simulink library "ADRC_Toolbox"  (R2024a)
settings: Solver=VariableStepAuto  StartTime=0.0  StopTime=10.0  RelTol=1e-3
undefined symbols (not defined in the file or in its folder): build_robot_screw, ToolGroup, ToolSet, Ts, x0
libraries: $bdroot x14, simulink x7
(part 1 of 2)
settings Model: Creator=91015  LastModifiedBy=Chenfei Wang
settings SolverCC: AlgebraicLoopSolver=TrustRegion
settings DebuggingCC: UnconnectedInputMsg=warning  UnconnectedOutputMsg=warning  UnconnectedLineMsg=warning
settings ModelReferenceCC: EnableRefExpFcnMdlSchedulingChecks=on
settings SFSimCC: CustomCodeUndefinedFunction=UseInterfaceOnly
settings RTWCC: GPUComputeCapability=3.5  DLArmComputeVersion=19.05

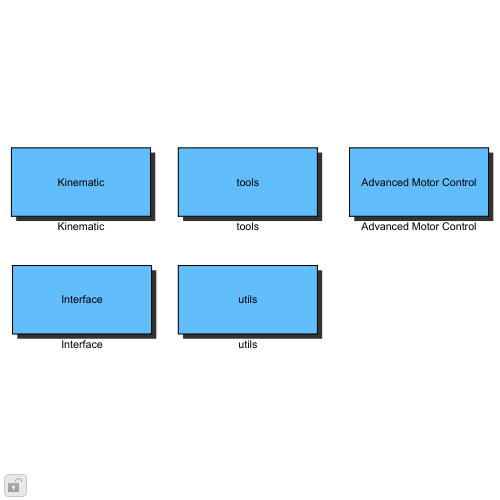
[thumbnail: Simulink's stored preview of the top-level diagram]
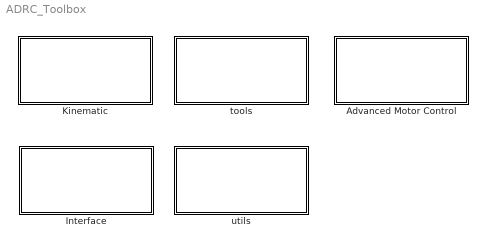
== system ADRC_Toolbox ==
  Advanced Motor Control : Subsystem  mask(tools){}
      mask Display: disp(get_param(gcb,'name'))
  Interface : Subsystem
      mask Display: disp(get_param(gcb,'name'))
  Kinematic : Subsystem
      mask Display: disp(get_param(gcb,'name'))
  tools : Subsystem  mask(tools){}
      mask Display: disp(get_param(gcb,'name'))
  utils : Subsystem  mask(tools){}
      mask Display: disp(get_param(gcb,'name'))

== system ADRC_Toolbox/Advanced Motor Control ==
  Basic : Subsystem
      mask Display: disp(get_param(gcb,'name'))
  Controller : Subsystem
      mask Display: disp(get_param(gcb,'name'))
  TD : Subsystem
      mask Display: disp(get_param(gcb,'name'))

== system ADRC_Toolbox/Interface ==
  note: encoder与 physical接口
  SC PC concat : Subsystem
  Tool Select : Subsystem
  allocateAllHands : MATLAB Function  TreatAsAtomicUnit=on
  checkToolTypeMatched : MATLAB Function  TreatAsAtomicUnit=on
  encoder2physical_PC : MATLAB Function  TreatAsAtomicUnit=on
  encoder2physical_SC : MATLAB Function  TreatAsAtomicUnit=on
  physical2encoder_PC : MATLAB Function  TreatAsAtomicUnit=on
  physical2encoder_SC : MATLAB Function  TreatAsAtomicUnit=on

== system ADRC_Toolbox/Kinematic ==
  Forward Kinematic : Subsystem  mask{ScrewObj=build_robot_screw, source_idx=0, target_idx=5}
      mask init:
      | ScrewObjName = get_param(gcb, 'ScrewObj');
      mask DialogControl DescGroupVar Prompt: Forward Kinematic
      mask DialogControl DescTextVar Prompt: 正向运动学,根据ScrewObj对象计算变换矩阵
      mask Display:
      | color('blue')
      | text(0.99, 0.99, ScrewObjName, 'horizontalAlignment', 'right', 'verticalAlignment','top');
      | 
      | color('black')
      | SourceText = ['Source: ' get_param(gcb,'source_idx')];
      | TargetText = ['Target: ' get_param(gcb,'target_idx')];
      | DescText = [SourceText newline TargetText];
      | text(0.5, 0.05, DescText, 'Interpreter', 'tex',  'horizontalAlignment', 'center','verticalAlignment','bottom');
      | 
      | color('black')
      | DescText = ['T' get_param(gcb,'source_idx') get_param(gcb,'target_idx')];
      | text(0.5, 0.8, DescText, 'Interpreter', 'tex',  'horizontalAlignment', 'center','verticalAlignment','bottom');
      | 
      | 
      | color('black')
      | port_label('input', 1, 'Config')
      | port_label('output', 1, 'Transform')
  Inverse Kinematic : Subsystem  mask{ScrewObj=build_robot_screw, Eomg=1e-5, Ev=1e-5, Lambda=0.2}
      mask init:
      | ScrewObjName = get_param(gcb, 'ScrewObj');
      mask DialogControl DescGroupVar Prompt: Inverse Kinematic
      mask DialogControl DescTextVar Prompt: 逆向运动学,给定T(相对base),使用LM算法求解
      mask Display:
      | color('blue')
      | text(0.99, 0.99, ScrewObjName, 'horizontalAlignment', 'right', 'verticalAlignment','top');
      | 
      | 
      | 
      | color('black')
      | port_label('input', 1, 'T')
      | port_label('input', 2, 'InitialGuass')
      | port_label('output', 1, 'theta')
      | port_label('output', 2, 'success')

== system ADRC_Toolbox/tools ==
  Clamp Tmatrix : MATLAB Function  TreatAsAtomicUnit=on
  Knife Tmatrix : MATLAB Function  TreatAsAtomicUnit=on
  Normal Tool Tmatrix : MATLAB Function  TreatAsAtomicUnit=on
  NormalTool_T2 : MATLAB Function  TreatAsAtomicUnit=on
  Scope Tmatrix : MATLAB Function  TreatAsAtomicUnit=on
  Screenangle2T : MATLAB Function  TreatAsAtomicUnit=on
  Stapler Tmatrix : MATLAB Function  TreatAsAtomicUnit=on
  ToolSet Select : Subsystem

== system ADRC_Toolbox/utils ==
  note: 错误代码
  Error Merge : Subsystem
  Error Store Memery : DataStoreMemory  DataStoreName=ErrorMemery  ReadBeforeWriteMsg=warning  WriteAfterWriteMsg=warning  WriteAfterReadMsg=warning  ShowAdditionalParam=off  OutDataTypeStr=uint16  Dimensions=1
  Tform2Vec : Subsystem
      mask Display:
      | color('black')
      | port_label('input', 1, 'T')
      | port_label('output', 1, 'Eul_ZYX')
      | port_label('output', 2, 'p')
  Tform2p : MATLAB Function  TreatAsAtomicUnit=on

== system ADRC_Toolbox/Advanced Motor Control/Basic ==
  Discrete State space with reset : Subsystem
      mask Display:
      | % port_label('input', 1, 'u')
      | % port_label('input', 2, 'A')
      | % port_label('input', 3, 'B')
      | % port_label('input', 4, 'C')
      | % port_label('input', 5, 'D')
      | % port_label('input', 6, 'x0')
      | % port_label('output', 1, 'y')
      | % port_label('output', 2, 'x')
      | % port_label('output', 3, 'dx')
      | 
      | text(0.5,0.65,'x_{k+1} = A x_k + B u_k',...
      |    'horizontalAlignment', 'center','texmode','on')
      | text(0.5,0.45,'y_k = C x_k + D u_k',...
      |    'horizontalAlignment', 'center','texmode','on')
      | text(0.5,0.25,'x0 with reset',...
      |    'horizontalAlignment', 'center','texmode','on')
  ODE4 Continue State space : Subsystem  mask{Ts=Ts}
      mask Display:
      | % port_label('input', 1, 'u')
      | % port_label('input', 2, 'A')
      | % port_label('input', 3, 'B')
      | % port_label('input', 4, 'C')
      | % port_label('input', 5, 'D')
      | % port_label('input', 6, 'x0')
      | % port_label('output', 1, 'y')
      | % port_label('output', 2, 'x')
      | % port_label('output', 3, 'dx')
      | 
      | text(0.5,0.65,'dx = A x + B u',...
      |    'horizontalAlignment', 'center','texmode','on')
      | text(0.5,0.45,'y = C x + D u',...
      |    'horizontalAlignment', 'center','texmode','on')
      | text(0.5,0.25,'x0 with reset',...
      |    'horizontalAlignment', 'center','texmode','on')
  State space with reset : Subsystem
      mask Display:
      | % port_label('input', 1, 'u')
      | % port_label('input', 2, 'A')
      | % port_label('input', 3, 'B')
      | % port_label('input', 4, 'C')
      | % port_label('input', 5, 'D')
      | % port_label('input', 6, 'x0')
      | % port_label('output', 1, 'y')
      | % port_label('output', 2, 'x')
      | % port_label('output', 3, 'dx')
      | 
      | text(0.5,0.65,'dx = A x + B u',...
      |    'horizontalAlignment', 'center','texmode','on')
      | text(0.5,0.45,'y = C x + D u',...
      |    'horizontalAlignment', 'center','texmode','on')
      | text(0.5,0.25,'x0 with reset',...
      |    'horizontalAlignment', 'center','texmode','on')

== system ADRC_Toolbox/Advanced Motor Control/Controller ==
  note: support code generation
  2nd order Discrete LADRC : Subsystem  mask{Ts=1e-3}
      mask prompts: Ts "Sampling Time"
  2nd order LADRC : Subsystem
  2nd order MC-ADRC : Subsystem  mask{a1=0}
      mask Display:
      | text(0.5,0.5,'ddx+a_1dx=b(u-f_{ext})',...
      |    'horizontalAlignment', 'center','texmode','on')
      | text(0.5,0.4,'u_{out}=u+f_{ext}',...
      |    'horizontalAlignment', 'center','texmode','on')
  LADRC 2nd : Subsystem  mask{wc=10, wo=50, b0=1, sat=[-1 1]}

== system ADRC_Toolbox/Advanced Motor Control/TD ==
  note: 带CBF约束2阶TD
  LTD template : Subsystem
  order2_LTD : Subsystem
  order2_LTD with damping : Subsystem
  order2_LTD with speed acc limit : Subsystem  mask{T=1e-2}
  order2_LTD with speed limit : Subsystem  mask{T=1e-2}
  order3_LTD : Subsystem
  "order5_LTD " : Subsystem
  order7_LTD : Subsystem
  order9_LTD : Subsystem

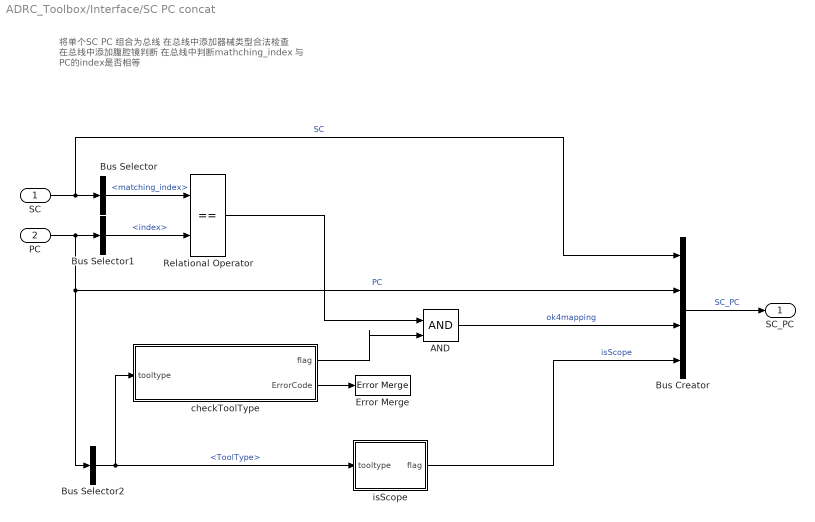
== system ADRC_Toolbox/Interface/SC PC concat ==
  note: 将单个SC PC 组合为总线
      | 在总线中添加器械类型合法检查
      | 在总线中添加腹腔镜判断
      | 在总线中判断mathching_index 与 PC的index是否相等
  SC : Inport  OutDataTypeStr=Bus: Hand_Bus
  PC : Inport  Port=2  OutDataTypeStr=Bus: Arm_Bus
  AND : Logic  IconShape=distinctive  AllPortsSameDT=off  OutDataTypeStr=boolean
  Bus Creator : BusCreator  Inputs=4
  Bus Selector : BusSelector  OutputSignals=matching_index
  Bus Selector1 : BusSelector  OutputSignals=index
  Bus Selector2 : BusSelector  OutputSignals=ToolType
  Error Merge : $bdroot/utils/Error Merge  SystemSampleTime=-1  VariantActivationTime=update diagram  AllowFlexibleInterface=on  Latency=0  AutoFrameSizeCalculation=off
  Relational Operator : RelationalOperator  Operator===  OutDataTypeStr=boolean  RndMeth=Simplest  InputSameDT=off
  checkToolType : MATLAB Function  TreatAsAtomicUnit=on
  isScope : MATLAB Function  TreatAsAtomicUnit=on
  SC_PC : Outport
  wires:
  Bus Selector1/1 -> Relational Operator/2  "<index>"
  isScope/1(flag) -> Bus Creator/4  "isScope"
  checkToolType/2(ErrorCode) -> Error Merge/1
  checkToolType/1(flag) -> AND/2
  SC/1 -> Bus Creator/1, Bus Selector/1  "SC"
  Relational Operator/1 -> AND/1
  AND/1 -> Bus Creator/3  "ok4mapping"
  Bus Creator/1 -> SC_PC/1  "SC_PC"
  Bus Selector/1 -> Relational Operator/1  "<matching_index>"
  Bus Selector2/1 -> checkToolType/1(tooltype), isScope/1(tooltype)  "<ToolType>"
  PC/1 -> Bus Creator/2, Bus Selector2/1, Bus Selector1/1  "PC"

== system ADRC_Toolbox/Interface/Tool Select ==
  index : Inport
  Bus Selector1 : BusSelector  OutputSignals=Tool1,Tool2,Tool3,Tool4
  Constant : Constant  Value=ToolSet  OutDataTypeStr=Bus: ToolSet_Bus
  Multiport Switch : MultiPortSwitch  DataPortOrder=Specify indices  DataPortIndices={1,2,3,4}  DiagnosticForDefault=None  SaturateOnIntegerOverflow=off  InputSameDT=off
  General Tool Config : Outport  OutDataTypeStr=Bus: GeneralTool_config_Bus
  wires:
  Constant/1 -> Bus Selector1/1
  Bus Selector1/4 -> Multiport Switch/5  "<Tool4>"
  Bus Selector1/2 -> Multiport Switch/3  "<Tool2>"
  Bus Selector1/1 -> Multiport Switch/2  "<Tool1>"
  Bus Selector1/3 -> Multiport Switch/4  "<Tool3>"
  Multiport Switch/1 -> General Tool Config/1
  index/1 -> Multiport Switch/1

== system ADRC_Toolbox/Kinematic/Forward Kinematic ==
  theta : Inport
  MATLAB System : MATLABSystem  System=ForwardKinematic_subs  screw=ScrewObj  SourceFrame=source_idx  TargetFrame=target_idx  SimulateUsing=Code generation
      mask Type: ForwardKinematic_subs
      mask Display:
      | disp('ForwardKinematic_subs');
      | port_label('input',1,'theta');
      | port_label('output',1,'T');
  Reshape : Reshape
  T : Outport  VectorParamsAs1DForOutWhenUnconnected=off
  wires:
  theta/1 -> Reshape/1
  Reshape/1 -> MATLAB System/1
  MATLAB System/1 -> T/1

== system ADRC_Toolbox/Kinematic/Inverse Kinematic ==
  T : Inport
  InitialGuass : Inport  Port=2
  MATLAB System : MATLABSystem  System=InverseKinematic_subs  screw=ScrewObj  eomg=Eomg  ev=Ev  lambda=Lambda  SimulateUsing=Code generation
      mask Type: InverseKinematic_subs
      mask Display:
      | disp('InverseKinematic_subs');
      | port_label('input',1,'T');
      | port_label('input',2,'theta0');
      | port_label('output',1,'theta');
      | port_label('output',2,'success');
  Reshape1 : Reshape
  Reshape2 : Reshape
  config : Outport  VectorParamsAs1DForOutWhenUnconnected=off
  sucess : Outport  Port=2  VectorParamsAs1DForOutWhenUnconnected=off
  wires:
  MATLAB System/2 -> sucess/1
  T/1 -> MATLAB System/1
  MATLAB System/1 -> Reshape2/1
  InitialGuass/1 -> Reshape1/1
  Reshape1/1 -> MATLAB System/2
  Reshape2/1 -> config/1

== system ADRC_Toolbox/tools/ToolSet Select ==
  index : Inport
  Bus Selector3 : BusSelector  OutputSignals=ToolSet1,ToolSet2,ToolSet3,ToolSet4
  Constant : Constant  Value=ToolGroup  OutDataTypeStr=Bus: ToolGroup_Bus
  Multiport Switch : MultiPortSwitch  DataPortOrder=Specify indices  DataPortIndices={1,2,3,4}  SaturateOnIntegerOverflow=off  InputSameDT=off
  ToolSet : Outport  OutDataTypeStr=Bus: ToolSet_Bus  VectorParamsAs1DForOutWhenUnconnected=off
  wires:
  Constant/1 -> Bus Selector3/1
  Bus Selector3/3 -> Multiport Switch/4  "<ToolSet3>"
  Bus Selector3/4 -> Multiport Switch/5  "<ToolSet4>"
  Bus Selector3/1 -> Multiport Switch/2  "<ToolSet1>"
  index/1 -> Multiport Switch/1
  Bus Selector3/2 -> Multiport Switch/3  "<ToolSet2>"
  Multiport Switch/1 -> ToolSet/1

== system ADRC_Toolbox/utils/Error Merge ==
  ErrorCode : Inport
  Data Type Conversion : DataTypeConversion  OutDataTypeStr=uint16  SaturateOnIntegerOverflow=off  RndMeth=Floor
  Error Merge : Stateflow chart  TreatAsAtomicUnit=on
  wires:
  ErrorCode/1 -> Data Type Conversion/1
  Data Type Conversion/1 -> Error Merge/1(ErrorCode)

== system ADRC_Toolbox/utils/Tform2Vec ==
  T : Inport  PortDimensions=[4,4]
  Reshape : Reshape
  Reshape1 : Reshape
  Tform2Vec : MATLAB Function  TreatAsAtomicUnit=on
  Eul : Outport  PortDimensions=3  VectorParamsAs1DForOutWhenUnconnected=off
  p : Outport  Port=2  PortDimensions=3  VectorParamsAs1DForOutWhenUnconnected=off
  wires:
  Reshape1/1 -> p/1
  Reshape/1 -> Eul/1
  Tform2Vec/2(p) -> Reshape1/1
  T/1 -> Tform2Vec/1(T)
  Tform2Vec/1(eul_angle) -> Reshape/1

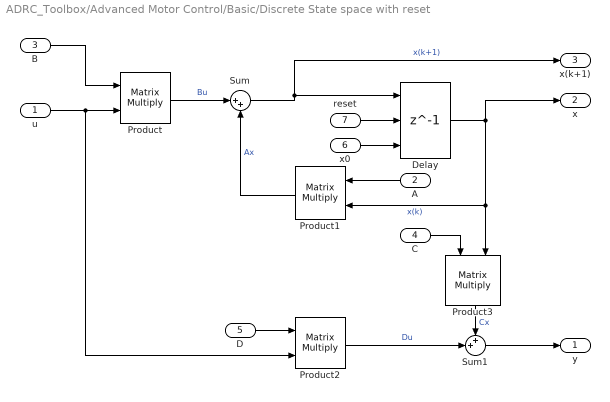
== system ADRC_Toolbox/Advanced Motor Control/Basic/Discrete State space with reset ==
  u : Inport
  A : Inport  Port=2
  B : Inport  Port=3
  C : Inport  Port=4
  D : Inport  Port=5
  x0 : Inport  Port=6
  reset : Inport  Port=7
  Delay : Delay  DelayLength=1  InitialConditionSource=Input port  ExternalReset=Rising
      settings: InputPortMap=u0,r5,p4
  Product{,1..3} (4 alike) : Product  SCDEnableBlockLinearizationSpecification=on  Multiplication=Matrix(*)
  Sum : Sum  Inputs=|++
  Sum1 : Sum  Inputs=++|
  y : Outport  VectorParamsAs1DForOutWhenUnconnected=off
  x : Outport  Port=2  VectorParamsAs1DForOutWhenUnconnected=off
  x(k+1) : Outport  Port=3  VectorParamsAs1DForOutWhenUnconnected=off
  wires:
  Product/1 -> Sum/1  "Bu"
  Sum/1 -> x(k+1)/1, Delay/1  "x(k+1)"
  B/1 -> Product/1
  Sum1/1 -> y/1
  Delay/1 -> x/1, Product3/2, Product1/2  "x(k)"
  D/1 -> Product2/1
  Product3/1 -> Sum1/1  "Cx"
  u/1 -> Product/2, Product2/2
  Product2/1 -> Sum1/2  "Du"
  Product1/1 -> Sum/2  "Ax"
  C/1 -> Product3/1
  A/1 -> Product1/1
  x0/1 -> Delay/3
  reset/1 -> Delay/2

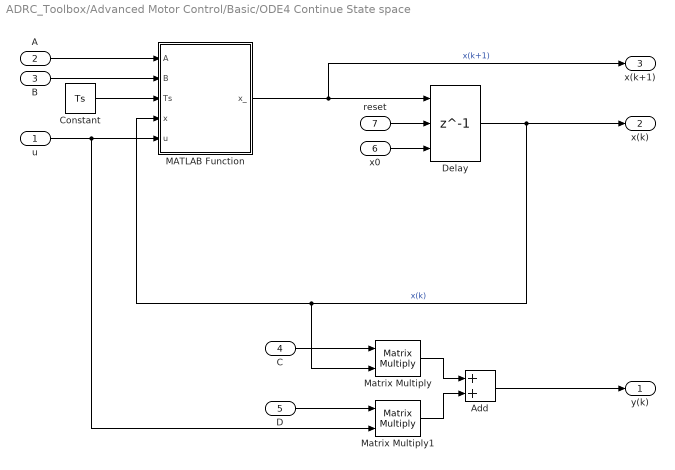
== system ADRC_Toolbox/Advanced Motor Control/Basic/ODE4 Continue State space ==
  u : Inport
  A : Inport  Port=2
  B : Inport  Port=3
  C : Inport  Port=4
  D : Inport  Port=5
  x0 : Inport  Port=6
  reset : Inport  Port=7
  Add : Sum
  Constant : Constant  Value=Ts
  Delay : Delay  DelayLength=1  InitialConditionSource=Input port  ExternalReset=Rising
      settings: InputPortMap=u0,r5,p4
  MATLAB Function : MATLAB Function  TreatAsAtomicUnit=on
  Matrix Multiply : Product  Multiplication=Matrix(*)
  Matrix Multiply1 : Product  Multiplication=Matrix(*)
  y(k) : Outport  VectorParamsAs1DForOutWhenUnconnected=off
  x(k) : Outport  Port=2  VectorParamsAs1DForOutWhenUnconnected=off
  x(k+1) : Outport  Port=3  VectorParamsAs1DForOutWhenUnconnected=off
  wires:
  Delay/1 -> Matrix Multiply/2, MATLAB Function/4(x), x(k)/1  "x(k)"
  x0/1 -> Delay/3
  reset/1 -> Delay/2
  MATLAB Function/1(x_) -> x(k+1)/1, Delay/1  "x(k+1)"
  A/1 -> MATLAB Function/1(A)
  B/1 -> MATLAB Function/2(B)
  Constant/1 -> MATLAB Function/3(Ts)
  u/1 -> Matrix Multiply1/2, MATLAB Function/5(u)
  C/1 -> Matrix Multiply/1
  D/1 -> Matrix Multiply1/1
  Matrix Multiply/1 -> Add/1
  Matrix Multiply1/1 -> Add/2
  Add/1 -> y(k)/1

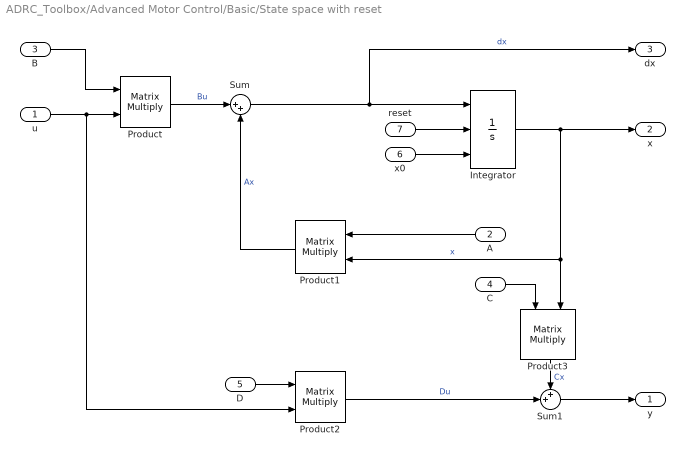
== system ADRC_Toolbox/Advanced Motor Control/Basic/State space with reset ==
  u : Inport
  A : Inport  Port=2
  B : Inport  Port=3
  C : Inport  Port=4
  D : Inport  Port=5
  x0 : Inport  Port=6
  reset : Inport  Port=7
  Integrator : Integrator  ExternalReset=rising  InitialConditionSource=external  InitialCondition=x0
  Product{,1..3} (4 alike) : Product  SCDEnableBlockLinearizationSpecification=on  Multiplication=Matrix(*)
  Sum : Sum  Inputs=|++
  Sum1 : Sum  Inputs=++|
  y : Outport  VectorParamsAs1DForOutWhenUnconnected=off
  x : Outport  Port=2  VectorParamsAs1DForOutWhenUnconnected=off
  dx : Outport  Port=3  VectorParamsAs1DForOutWhenUnconnected=off
  wires:
  x0/1 -> Integrator/3
  Product/1 -> Sum/1  "Bu"
  Sum/1 -> dx/1, Integrator/1  "dx"
  A/1 -> Product1/1
  u/1 -> Product/2, Product2/2
  Product1/1 -> Sum/2  "Ax"
  D/1 -> Product2/1
  Product3/1 -> Sum1/1  "Cx"
  B/1 -> Product/1
  Integrator/1 -> Product3/2, Product1/2, x/1  "x"
  Sum1/1 -> y/1
  Product2/1 -> Sum1/2  "Du"
  C/1 -> Product3/1
  reset/1 -> Integrator/2

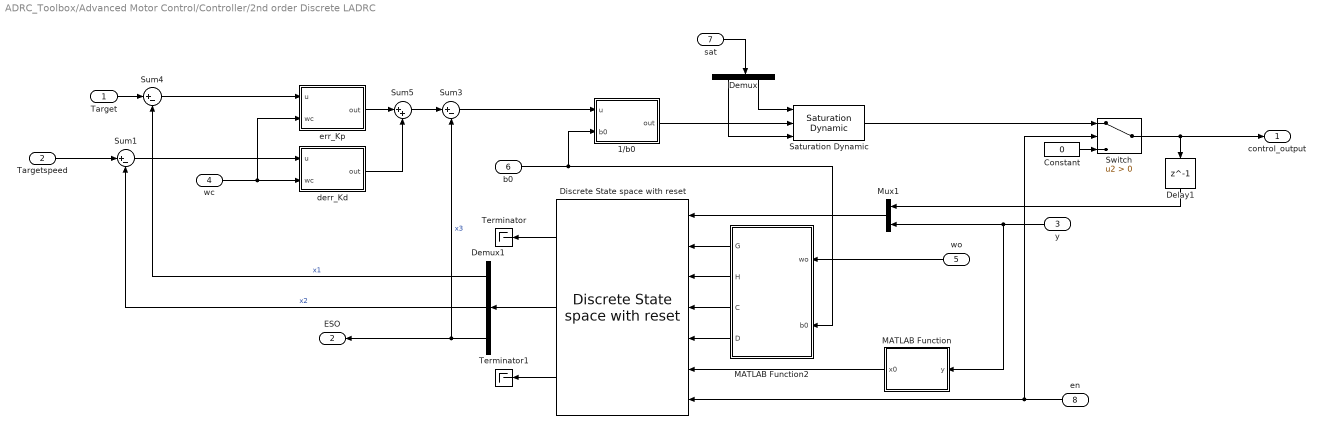
== system ADRC_Toolbox/Advanced Motor Control/Controller/2nd order Discrete LADRC ==
  Target : Inport  PortDimensions=1
  Targetspeed : Inport  Port=2  PortDimensions=1
  y : Inport  Port=3  PortDimensions=1
  wc : Inport  Port=4  PortDimensions=1
  wo : Inport  Port=5  PortDimensions=1
  b0 : Inport  Port=6  PortDimensions=1
  sat : Inport  Port=7  PortDimensions=2
  en : Inport  Port=8  PortDimensions=1
  1/b0 : MATLAB Function  TreatAsAtomicUnit=on
  Constant : Constant  Value=0
  Delay1 : Delay  DelayLength=1  InitialCondition=0
  Demux : Demux  Outputs=2
  Demux1 : Demux  Outputs=3
  Discrete State space with reset : $bdroot/Advanced Motor Control/Basic/Discrete State space with reset  SystemSampleTime=-1  VariantActivationTime=update diagram  AllowFlexibleInterface=on  Latency=0  AutoFrameSizeCalculation=off
  MATLAB Function : MATLAB Function  TreatAsAtomicUnit=on
  MATLAB Function2 : MATLAB Function  TreatAsAtomicUnit=on
  Mux1 : Mux  Inputs=2
  Saturation Dynamic : simulink/Discontinuities/Saturation Dynamic  OutMin=[]  OutMax=[]  OutDataTypeStr=Inherit: Same as second input  OutDataType=fixdt(1, 16)  OutScaling=2^-10  DoSatur=off
  Sum1 : Sum  Inputs=|+-
  Sum3 : Sum  Inputs=|+-
  Sum4 : Sum  Inputs=|+-
  Sum5 : Sum  Inputs=|++
  Switch : Switch  Criteria=u2 > Threshold  SaturateOnIntegerOverflow=off  InputSameDT=off
  Terminator : Terminator
  Terminator1 : Terminator
  derr_Kd : MATLAB Function  TreatAsAtomicUnit=on
  err_Kp : MATLAB Function  TreatAsAtomicUnit=on
  control_output : Outport  VectorParamsAs1DForOutWhenUnconnected=off
  ESO : Outport  Port=2
  wires:
  Switch/1 -> Delay1/1, control_output/1
  MATLAB Function/1(x0) -> Discrete State space with reset/6
  Delay1/1 -> Mux1/1
  sat/1 -> Demux/1
  Demux/2 -> Saturation Dynamic/1
  Demux/1 -> Saturation Dynamic/3
  Target/1 -> Sum4/1
  Sum4/1 -> err_Kp/1(u)
  Demux1/1 -> Sum4/2  "x1"
  Mux1/1 -> Discrete State space with reset/1
  MATLAB Function2/2(H) -> Discrete State space with reset/3
  1/b0/1(out) -> Saturation Dynamic/2
  MATLAB Function2/4(D) -> Discrete State space with reset/5
  MATLAB Function2/1(G) -> Discrete State space with reset/2
  Sum5/1 -> Sum3/1
  y/1 -> MATLAB Function/1(y), Mux1/2
  derr_Kd/1(out) -> Sum5/2
  err_Kp/1(out) -> Sum5/1
  Sum3/1 -> 1/b0/1(u)
  MATLAB Function2/3(C) -> Discrete State space with reset/4
  wo/1 -> MATLAB Function2/1(wo)
  Demux1/3 -> ESO/1, Sum3/2  "x3"
  b0/1 -> MATLAB Function2/2(b0), 1/b0/2(b0)
  wc/1 -> err_Kp/2(wc), derr_Kd/2(wc)
  Targetspeed/1 -> Sum1/1
  Demux1/2 -> Sum1/2  "x2"
  Sum1/1 -> derr_Kd/1(u)
  Discrete State space with reset/1 -> Terminator/1
  Saturation Dynamic/1 -> Switch/1
  en/1 -> Discrete State space with reset/7, Switch/2
  Constant/1 -> Switch/3
  Discrete State space with reset/2 -> Demux1/1
  Discrete State space with reset/3 -> Terminator1/1

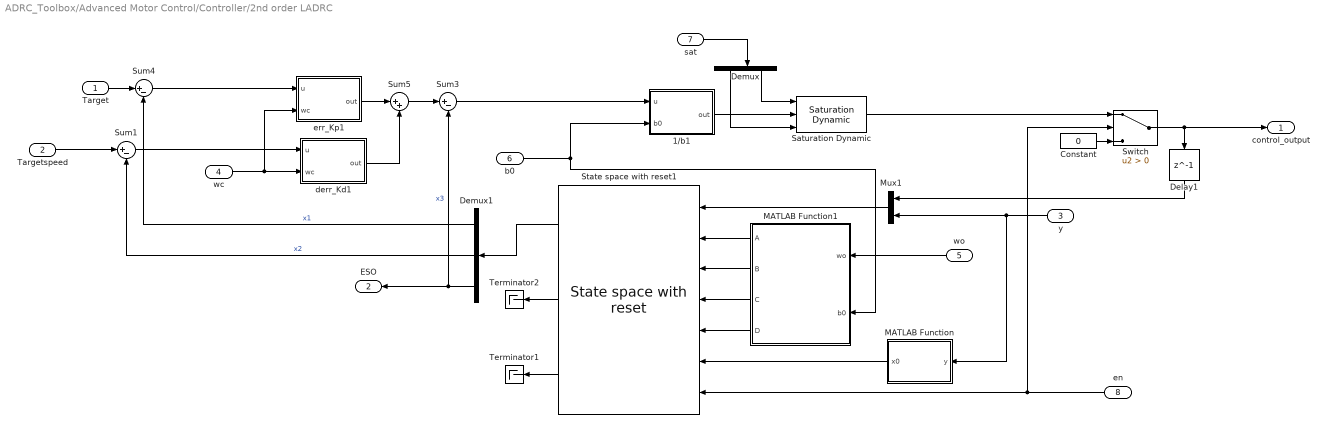
== system ADRC_Toolbox/Advanced Motor Control/Controller/2nd order LADRC ==
  Target : Inport  PortDimensions=1
  Targetspeed : Inport  Port=2  PortDimensions=1
  y : Inport  Port=3  PortDimensions=1
  wc : Inport  Port=4  PortDimensions=1
  wo : Inport  Port=5  PortDimensions=1
  b0 : Inport  Port=6  PortDimensions=1
  sat : Inport  Port=7  PortDimensions=2
  en : Inport  Port=8  PortDimensions=1
  1/b1 : MATLAB Function  TreatAsAtomicUnit=on
  Constant : Constant  Value=0
  Delay1 : Delay  DelayLength=1  InitialCondition=0
  Demux : Demux  Outputs=2
  Demux1 : Demux  Outputs=3
  MATLAB Function : MATLAB Function  TreatAsAtomicUnit=on
  MATLAB Function1 : MATLAB Function  TreatAsAtomicUnit=on
  Mux1 : Mux  Inputs=2
  Saturation Dynamic : simulink/Discontinuities/Saturation Dynamic  OutMin=[]  OutMax=[]  OutDataTypeStr=Inherit: Same as second input  OutDataType=fixdt(1, 16)  OutScaling=2^-10  DoSatur=off
  State space with reset1 : $bdroot/Advanced Motor Control/Basic/State space with reset  SystemSampleTime=-1  VariantActivationTime=update diagram  AllowFlexibleInterface=on  Latency=0  AutoFrameSizeCalculation=off
  Sum1 : Sum  Inputs=|+-
  Sum3 : Sum  Inputs=|+-
  Sum4 : Sum  Inputs=|+-
  Sum5 : Sum  Inputs=|++
  Switch : Switch  Criteria=u2 > Threshold  SaturateOnIntegerOverflow=off  InputSameDT=off
  Terminator1 : Terminator
  Terminator2 : Terminator
  derr_Kd1 : MATLAB Function  TreatAsAtomicUnit=on
  err_Kp1 : MATLAB Function  TreatAsAtomicUnit=on
  control_output : Outport  VectorParamsAs1DForOutWhenUnconnected=off
  ESO : Outport  Port=2
  wires:
  Switch/1 -> Delay1/1, control_output/1
  MATLAB Function/1(x0) -> State space with reset1/6
  State space with reset1/1 -> Demux1/1
  Delay1/1 -> Mux1/1
  sat/1 -> Demux/1
  Demux/2 -> Saturation Dynamic/1
  Demux/1 -> Saturation Dynamic/3
  Target/1 -> Sum4/1
  Sum4/1 -> err_Kp1/1(u)
  Demux1/1 -> Sum4/2  "x1"
  Mux1/1 -> State space with reset1/1
  MATLAB Function1/2(B) -> State space with reset1/3
  1/b1/1(out) -> Saturation Dynamic/2
  MATLAB Function1/4(D) -> State space with reset1/5
  MATLAB Function1/1(A) -> State space with reset1/2
  Sum5/1 -> Sum3/1
  y/1 -> MATLAB Function/1(y), Mux1/2
  derr_Kd1/1(out) -> Sum5/2
  err_Kp1/1(out) -> Sum5/1
  Sum3/1 -> 1/b1/1(u)
  MATLAB Function1/3(C) -> State space with reset1/4
  wo/1 -> MATLAB Function1/1(wo)
  Demux1/3 -> ESO/1, Sum3/2  "x3"
  b0/1 -> MATLAB Function1/2(b0), 1/b1/2(b0)
  wc/1 -> derr_Kd1/2(wc), err_Kp1/2(wc)
  Targetspeed/1 -> Sum1/1
  Demux1/2 -> Sum1/2  "x2"
  Sum1/1 -> derr_Kd1/1(u)
  en/1 -> State space with reset1/7, Switch/2
  Saturation Dynamic/1 -> Switch/1
  Constant/1 -> Switch/3
  State space with reset1/3 -> Terminator1/1
  State space with reset1/2 -> Terminator2/1

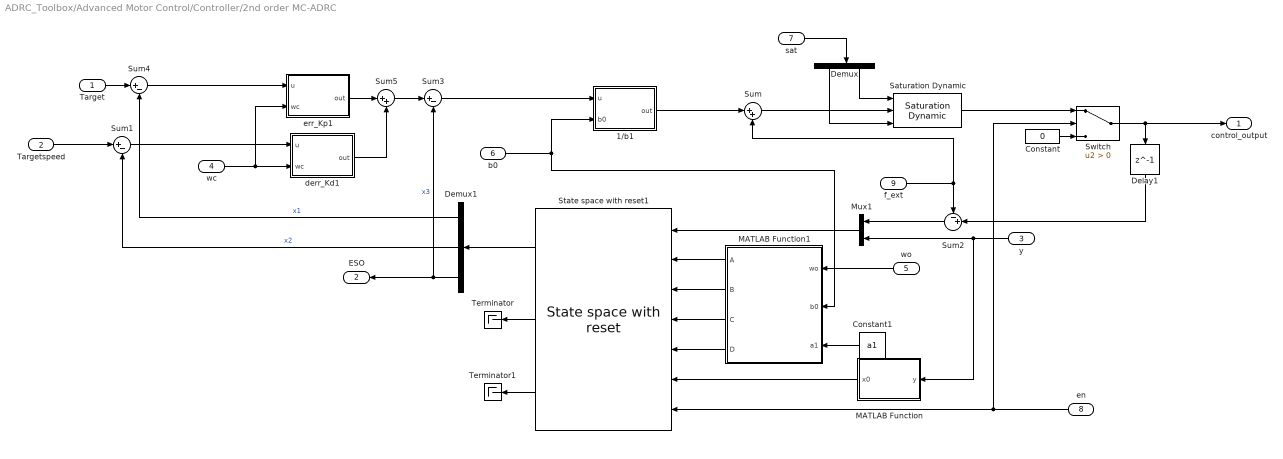
== system ADRC_Toolbox/Advanced Motor Control/Controller/2nd order MC-ADRC ==
  Target : Inport  PortDimensions=1
  Targetspeed : Inport  Port=2  PortDimensions=1
  y : Inport  Port=3  PortDimensions=1
  wc : Inport  Port=4  PortDimensions=1
  wo : Inport  Port=5  PortDimensions=1
  b0 : Inport  Port=6  PortDimensions=1
  sat : Inport  Port=7  PortDimensions=2
  en : Inport  Port=8  PortDimensions=1
  f_ext : Inport  Port=9
  1/b1 : MATLAB Function  TreatAsAtomicUnit=on
  Constant : Constant  Value=0
  Constant1 : Constant  Value=a1
  Delay1 : Delay  DelayLength=1  InitialCondition=0
  Demux : Demux  Outputs=2
  Demux1 : Demux  Outputs=3
  MATLAB Function : MATLAB Function  TreatAsAtomicUnit=on
  MATLAB Function1 : MATLAB Function  TreatAsAtomicUnit=on
  Mux1 : Mux  Inputs=2
  Saturation Dynamic : simulink/Discontinuities/Saturation Dynamic  OutMin=[]  OutMax=[]  OutDataTypeStr=Inherit: Same as second input  OutDataType=fixdt(1, 16)  OutScaling=2^-10  DoSatur=off
  State space with reset1 : $bdroot/Advanced Motor Control/Basic/State space with reset  SystemSampleTime=-1  VariantActivationTime=update diagram  AllowFlexibleInterface=on  Latency=0  AutoFrameSizeCalculation=off
  Sum : Sum  Inputs=|++
  Sum1 : Sum  Inputs=|+-
  Sum2 : Sum  Inputs=-+|
  Sum3 : Sum  Inputs=|+-
  Sum4 : Sum  Inputs=|+-
  Sum5 : Sum  Inputs=|++
  Switch : Switch  Criteria=u2 > Threshold  SaturateOnIntegerOverflow=off  InputSameDT=off
  Terminator : Terminator
  Terminator1 : Terminator
  derr_Kd1 : MATLAB Function  TreatAsAtomicUnit=on
  err_Kp1 : MATLAB Function  TreatAsAtomicUnit=on
  control_output : Outport  VectorParamsAs1DForOutWhenUnconnected=off
  ESO : Outport  Port=2
  wires:
  State space with reset1/3 -> Terminator1/1
  Constant/1 -> Switch/3
  Saturation Dynamic/1 -> Switch/1
  en/1 -> State space with reset1/7, Switch/2
  Sum1/1 -> derr_Kd1/1(u)
  Demux1/2 -> Sum1/2  "x2"
  Targetspeed/1 -> Sum1/1
  wc/1 -> err_Kp1/2(wc), derr_Kd1/2(wc)
  b0/1 -> 1/b1/2(b0), MATLAB Function1/2(b0)
  Demux1/3 -> ESO/1, Sum3/2  "x3"
  wo/1 -> MATLAB Function1/1(wo)
  MATLAB Function1/3(C) -> State space with reset1/4
  Sum3/1 -> 1/b1/1(u)
  err_Kp1/1(out) -> Sum5/1
  derr_Kd1/1(out) -> Sum5/2
  y/1 -> Mux1/2, MATLAB Function/1(y)
  Sum5/1 -> Sum3/1
  MATLAB Function1/1(A) -> State space with reset1/2
  MATLAB Function1/4(D) -> State space with reset1/5
  MATLAB Function1/2(B) -> State space with reset1/3
  Mux1/1 -> State space with reset1/1
  Demux1/1 -> Sum4/2  "x1"
  Sum4/1 -> err_Kp1/1(u)
  Target/1 -> Sum4/1
  Demux/1 -> Saturation Dynamic/3
  Demux/2 -> Saturation Dynamic/1
  sat/1 -> Demux/1
  State space with reset1/1 -> Demux1/1
  MATLAB Function/1(x0) -> State space with reset1/6
  Switch/1 -> control_output/1, Delay1/1
  Constant1/1 -> MATLAB Function1/3(a1)
  1/b1/1(out) -> Sum/1
  Sum/1 -> Saturation Dynamic/2
  f_ext/1 -> Sum/2, Sum2/1
  Delay1/1 -> Sum2/2
  Sum2/1 -> Mux1/1
  State space with reset1/2 -> Terminator/1

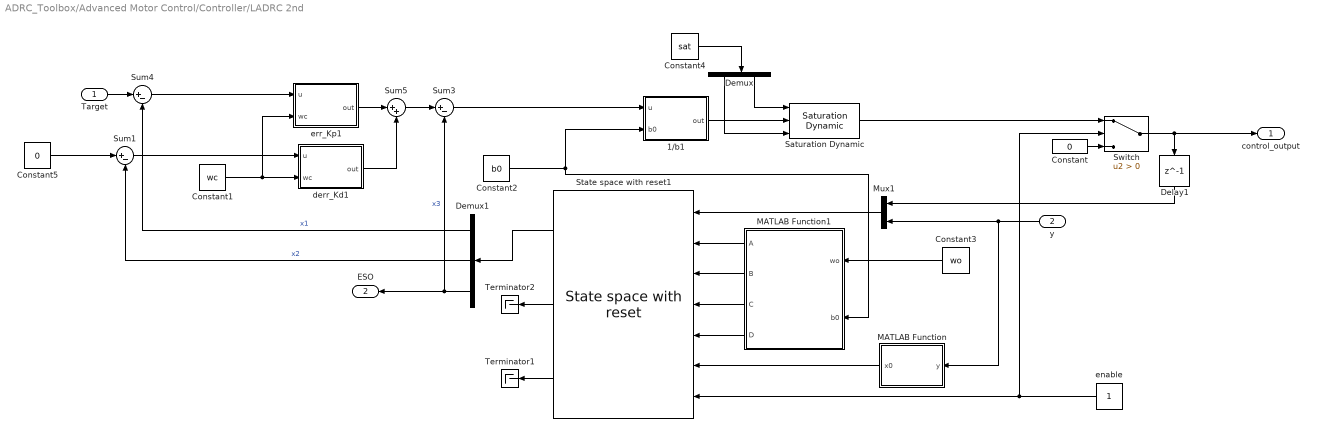
== system ADRC_Toolbox/Advanced Motor Control/Controller/LADRC 2nd ==
  Target : Inport  PortDimensions=1
  y : Inport  Port=2  PortDimensions=1
  1/b1 : MATLAB Function  TreatAsAtomicUnit=on
  Constant : Constant  Value=0
  Constant1 : Constant  Value=wc
  Constant2 : Constant  Value=b0
  Constant3 : Constant  Value=wo
  Constant4 : Constant  Value=sat
  Constant5 : Constant  Value=0
  Delay1 : Delay  DelayLength=1  InitialCondition=0
  Demux : Demux  Outputs=2
  Demux1 : Demux  Outputs=3
  MATLAB Function : MATLAB Function  TreatAsAtomicUnit=on
  MATLAB Function1 : MATLAB Function  TreatAsAtomicUnit=on
  Mux1 : Mux  Inputs=2
  Saturation Dynamic : simulink/Discontinuities/Saturation Dynamic  OutMin=[]  OutMax=[]  OutDataTypeStr=Inherit: Same as second input  OutDataType=fixdt(1, 16)  OutScaling=2^-10  DoSatur=off
  State space with reset1 : $bdroot/Advanced Motor Control/Basic/State space with reset  SystemSampleTime=-1  VariantActivationTime=update diagram  AllowFlexibleInterface=on  Latency=0  AutoFrameSizeCalculation=off
  Sum1 : Sum  Inputs=|+-
  Sum3 : Sum  Inputs=|+-
  Sum4 : Sum  Inputs=|+-
  Sum5 : Sum  Inputs=|++
  Switch : Switch  Criteria=u2 > Threshold  SaturateOnIntegerOverflow=off  InputSameDT=off
  Terminator1 : Terminator
  Terminator2 : Terminator
  derr_Kd1 : MATLAB Function  TreatAsAtomicUnit=on
  enable : Constant
  err_Kp1 : MATLAB Function  TreatAsAtomicUnit=on
  control_output : Outport  VectorParamsAs1DForOutWhenUnconnected=off
  ESO : Outport  Port=2
  wires:
  State space with reset1/2 -> Terminator2/1
  State space with reset1/3 -> Terminator1/1
  Constant/1 -> Switch/3
  Saturation Dynamic/1 -> Switch/1
  enable/1 -> Switch/2, State space with reset1/7
  Sum1/1 -> derr_Kd1/1(u)
  Demux1/2 -> Sum1/2  "x2"
  Constant5/1 -> Sum1/1
  Constant1/1 -> err_Kp1/2(wc), derr_Kd1/2(wc)
  Constant2/1 -> 1/b1/2(b0), MATLAB Function1/2(b0)
  Demux1/3 -> Sum3/2, ESO/1  "x3"
  Constant3/1 -> MATLAB Function1/1(wo)
  MATLAB Function1/3(C) -> State space with reset1/4
  Sum3/1 -> 1/b1/1(u)
  err_Kp1/1(out) -> Sum5/1
  derr_Kd1/1(out) -> Sum5/2
  y/1 -> Mux1/2, MATLAB Function/1(y)
  Sum5/1 -> Sum3/1
  MATLAB Function1/1(A) -> State space with reset1/2
  MATLAB Function1/4(D) -> State space with reset1/5
  1/b1/1(out) -> Saturation Dynamic/2
  MATLAB Function1/2(B) -> State space with reset1/3
  Mux1/1 -> State space with reset1/1
  Demux1/1 -> Sum4/2  "x1"
  Sum4/1 -> err_Kp1/1(u)
  Target/1 -> Sum4/1
  Demux/1 -> Saturation Dynamic/3
  Demux/2 -> Saturation Dynamic/1
  Constant4/1 -> Demux/1
  Delay1/1 -> Mux1/1
  State space with reset1/1 -> Demux1/1
  MATLAB Function/1(x0) -> State space with reset1/6
  Switch/1 -> control_output/1, Delay1/1

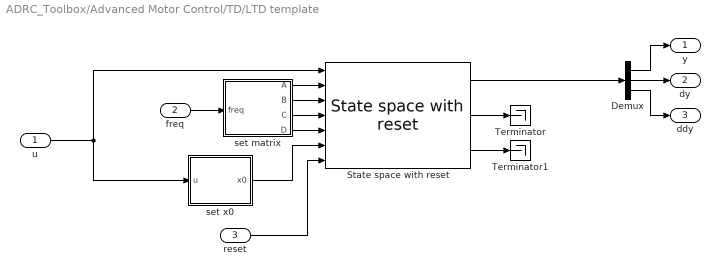
== system ADRC_Toolbox/Advanced Motor Control/TD/LTD template ==
  u : Inport
  freq : Inport  Port=2
  reset : Inport  Port=3
  Demux : Demux  Outputs=3
  State space with reset : $bdroot/Advanced Motor Control/Basic/State space with reset  SystemSampleTime=-1  VariantActivationTime=update diagram  AllowFlexibleInterface=on  Latency=0  AutoFrameSizeCalculation=off
  Terminator : Terminator
  Terminator1 : Terminator
  set matrix : MATLAB Function  TreatAsAtomicUnit=on
  set x0 : MATLAB Function  TreatAsAtomicUnit=on
  y : Outport  VectorParamsAs1DForOutWhenUnconnected=off
  dy : Outport  Port=2  VectorParamsAs1DForOutWhenUnconnected=off
  ddy : Outport  Port=3  VectorParamsAs1DForOutWhenUnconnected=off
  wires:
  set matrix/4(D) -> State space with reset/5
  set matrix/3(C) -> State space with reset/4
  freq/1 -> set matrix/1(freq)
  set matrix/1(A) -> State space with reset/2
  set matrix/2(B) -> State space with reset/3
  u/1 -> State space with reset/1, set x0/1(u)
  State space with reset/1 -> Demux/1
  Demux/1 -> y/1
  Demux/2 -> dy/1
  Demux/3 -> ddy/1
  State space with reset/2 -> Terminator/1
  State space with reset/3 -> Terminator1/1
  set x0/1(x0) -> State space with reset/6
  reset/1 -> State space with reset/7

== system ADRC_Toolbox/Advanced Motor Control/TD/order2_LTD ==
  u : Inport
  freq : Inport  Port=2
  reset : Inport  Port=3
  Demux : Demux  Outputs=2
  State space with reset : $bdroot/Advanced Motor Control/Basic/State space with reset  SystemSampleTime=-1  VariantActivationTime=update diagram  AllowFlexibleInterface=on  Latency=0  AutoFrameSizeCalculation=off
  Terminator : Terminator
  Terminator1 : Terminator
  set matrix : MATLAB Function  TreatAsAtomicUnit=on
  set x0 : MATLAB Function  TreatAsAtomicUnit=on
  y : Outport  VectorParamsAs1DForOutWhenUnconnected=off
  dy : Outport  Port=2  VectorParamsAs1DForOutWhenUnconnected=off
  wires:
  set matrix/4(D) -> State space with reset/5
  set matrix/3(C) -> State space with reset/4
  freq/1 -> set matrix/1(freq)
  set matrix/1(A) -> State space with reset/2
  set matrix/2(B) -> State space with reset/3
  u/1 -> State space with reset/1, set x0/1(u)
  State space with reset/1 -> Demux/1
  Demux/1 -> y/1
  Demux/2 -> dy/1
  State space with reset/2 -> Terminator/1
  State space with reset/3 -> Terminator1/1
  set x0/1(x0) -> State space with reset/6
  reset/1 -> State space with reset/7

== system ADRC_Toolbox/Advanced Motor Control/TD/order2_LTD with damping ==
  u : Inport
  freq : Inport  Port=2
  xi : Inport  Port=3
  reset : Inport  Port=4
  Demux : Demux  Outputs=2
  State space with reset : $bdroot/Advanced Motor Control/Basic/State space with reset  SystemSampleTime=-1  VariantActivationTime=update diagram  AllowFlexibleInterface=on  Latency=0  AutoFrameSizeCalculation=off
  Terminator : Terminator
  Terminator1 : Terminator
  set matrix : MATLAB Function  TreatAsAtomicUnit=on
  set x0 : MATLAB Function  TreatAsAtomicUnit=on
  y : Outport  VectorParamsAs1DForOutWhenUnconnected=off
  dy : Outport  Port=2  VectorParamsAs1DForOutWhenUnconnected=off
  wires:
  set matrix/4(D) -> State space with reset/5
  set matrix/3(C) -> State space with reset/4
  freq/1 -> set matrix/1(freq)
  set matrix/1(A) -> State space with reset/2
  set matrix/2(B) -> State space with reset/3
  u/1 -> State space with reset/1, set x0/1(u)
  State space with reset/1 -> Demux/1
  Demux/1 -> y/1
  Demux/2 -> dy/1
  State space with reset/2 -> Terminator/1
  State space with reset/3 -> Terminator1/1
  set x0/1(x0) -> State space with reset/6
  reset/1 -> State space with reset/7
  xi/1 -> set matrix/2(xi)

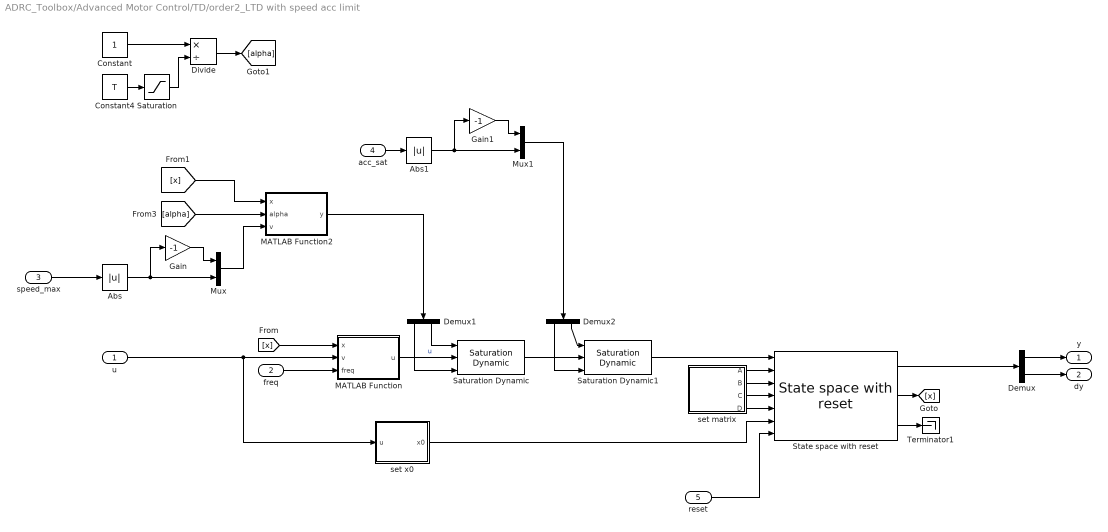
== system ADRC_Toolbox/Advanced Motor Control/TD/order2_LTD with speed acc limit ==
  u : Inport
  freq : Inport  Port=2
  speed_max : Inport  Port=3  PortDimensions=1
  acc_sat : Inport  Port=4  PortDimensions=1
  reset : Inport  Port=5
  Abs : Abs  SaturateOnIntegerOverflow=off
  Abs1 : Abs  SaturateOnIntegerOverflow=off
  Constant : Constant
  Constant4 : Constant  Value=T
  Demux : Demux  Outputs=2
  Demux1 : Demux  Outputs=2
  Demux2 : Demux  Outputs=2
  Divide : Product  Inputs=*/
  Gain : Gain  Gain=-1
  Gain1 : Gain  Gain=-1
  MATLAB Function : MATLAB Function  TreatAsAtomicUnit=on
  MATLAB Function2 : MATLAB Function  TreatAsAtomicUnit=on
  Mux : Mux  Inputs=2
  Mux1 : Mux  Inputs=2
  Saturation : Saturate  UpperLimit=1  LowerLimit=0.001
  Saturation Dynamic : simulink/Discontinuities/Saturation Dynamic  OutMin=[]  OutMax=[]  OutDataTypeStr=Inherit: Same as second input  OutDataType=fixdt(1, 16)  OutScaling=2^-10  DoSatur=off
  Saturation Dynamic1 : simulink/Discontinuities/Saturation Dynamic  OutMin=[]  OutMax=[]  OutDataTypeStr=Inherit: Same as second input  OutDataType=fixdt(1, 16)  OutScaling=2^-10  DoSatur=off
  State space with reset : $bdroot/Advanced Motor Control/Basic/State space with reset  SystemSampleTime=-1  VariantActivationTime=update diagram  AllowFlexibleInterface=on  Latency=0  AutoFrameSizeCalculation=off
  Terminator1 : Terminator
  set matrix : MATLAB Function  TreatAsAtomicUnit=on
  set x0 : MATLAB Function  TreatAsAtomicUnit=on
  y : Outport  VectorParamsAs1DForOutWhenUnconnected=off
  dy : Outport  Port=2  VectorParamsAs1DForOutWhenUnconnected=off
  wires:
  set matrix/4(D) -> State space with reset/5
  set matrix/3(C) -> State space with reset/4
  set matrix/1(A) -> State space with reset/2
  set matrix/2(B) -> State space with reset/3
  u/1 -> set x0/1(u), MATLAB Function/2(v)
  State space with reset/1 -> Demux/1
  Demux/1 -> y/1
  Demux/2 -> dy/1
  State space with reset/3 -> Terminator1/1
  set x0/1(x0) -> State space with reset/6
  reset/1 -> State space with reset/7
  freq/1 -> MATLAB Function/3(freq)
  MATLAB Function/1(u) -> Saturation Dynamic/2  "u"
  State space with reset/2 -> [x]
  [x] -> MATLAB Function/1(x)
  Constant4/1 -> Saturation/1
  Divide/1 -> [alpha]
  Constant/1 -> Divide/1
  Saturation/1 -> Divide/2
  Saturation Dynamic1/1 -> State space with reset/1
  Saturation Dynamic/1 -> Saturation Dynamic1/2
  Demux1/1 -> Saturation Dynamic/3
  Demux1/2 -> Saturation Dynamic/1
  Demux2/1 -> Saturation Dynamic1/3
  Demux2/2 -> Saturation Dynamic1/1
  Gain/1 -> Mux/1
  Abs/1 -> Gain/1, Mux/2
  speed_max/1 -> Abs/1
  [x] -> MATLAB Function2/1(x)
  [alpha] -> MATLAB Function2/2(alpha)
  Mux/1 -> MATLAB Function2/3(v)
  MATLAB Function2/1(y) -> Demux1/1
  Abs1/1 -> Gain1/1, Mux1/2
  Mux1/1 -> Demux2/1
  Gain1/1 -> Mux1/1
  acc_sat/1 -> Abs1/1

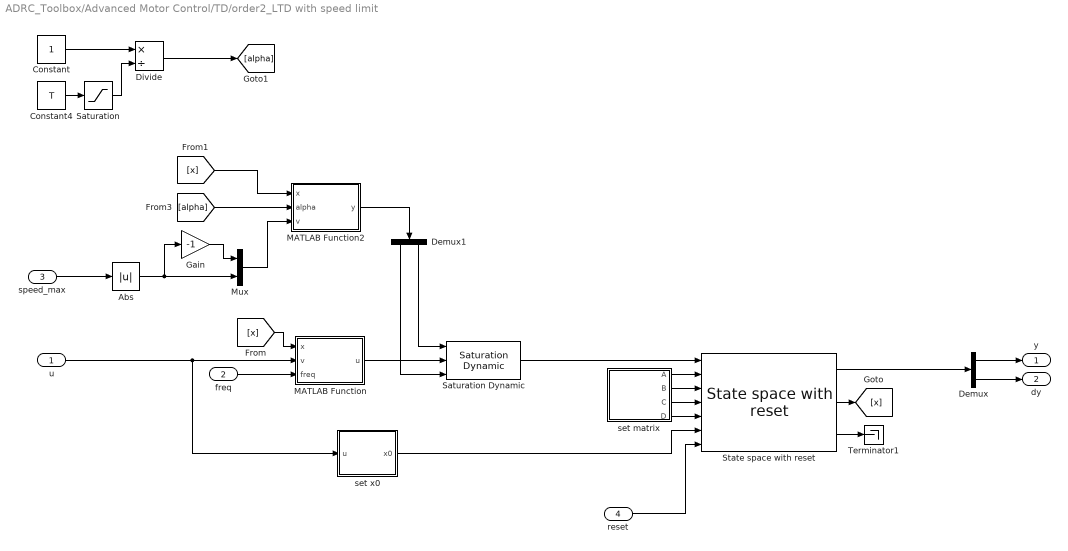
== system ADRC_Toolbox/Advanced Motor Control/TD/order2_LTD with speed limit ==
  u : Inport
  freq : Inport  Port=2
  speed_max : Inport  Port=3  PortDimensions=1
  reset : Inport  Port=4
  Abs : Abs  SaturateOnIntegerOverflow=off
  Constant : Constant
  Constant4 : Constant  Value=T
  Demux : Demux  Outputs=2
  Demux1 : Demux  Outputs=2
  Divide : Product  Inputs=*/
  Gain : Gain  Gain=-1
  MATLAB Function : MATLAB Function  TreatAsAtomicUnit=on
  MATLAB Function2 : MATLAB Function  TreatAsAtomicUnit=on
  Mux : Mux  Inputs=2
  Saturation : Saturate  UpperLimit=1  LowerLimit=0.001
  Saturation Dynamic : simulink/Discontinuities/Saturation Dynamic  OutMin=[]  OutMax=[]  OutDataTypeStr=Inherit: Same as second input  OutDataType=fixdt(1, 16)  OutScaling=2^-10  DoSatur=off
  State space with reset : $bdroot/Advanced Motor Control/Basic/State space with reset  SystemSampleTime=-1  VariantActivationTime=update diagram  AllowFlexibleInterface=on  Latency=0  AutoFrameSizeCalculation=off
  Terminator1 : Terminator
  set matrix : MATLAB Function  TreatAsAtomicUnit=on
  set x0 : MATLAB Function  TreatAsAtomicUnit=on
  y : Outport  VectorParamsAs1DForOutWhenUnconnected=off
  dy : Outport  Port=2  VectorParamsAs1DForOutWhenUnconnected=off
  wires:
  set matrix/4(D) -> State space with reset/5
  set matrix/3(C) -> State space with reset/4
  set matrix/1(A) -> State space with reset/2
  set matrix/2(B) -> State space with reset/3
  u/1 -> set x0/1(u), MATLAB Function/2(v)
  State space with reset/1 -> Demux/1
  Demux/1 -> y/1
  Demux/2 -> dy/1
  State space with reset/3 -> Terminator1/1
  set x0/1(x0) -> State space with reset/6
  reset/1 -> State space with reset/7
  freq/1 -> MATLAB Function/3(freq)
  MATLAB Function/1(u) -> Saturation Dynamic/2
  Saturation Dynamic/1 -> State space with reset/1
  State space with reset/2 -> [x]
  [x] -> MATLAB Function/1(x)
  [x] -> MATLAB Function2/1(x)
  [alpha] -> MATLAB Function2/2(alpha)
  Demux1/2 -> Saturation Dynamic/1
  Demux1/1 -> Saturation Dynamic/3
  MATLAB Function2/1(y) -> Demux1/1
  Constant4/1 -> Saturation/1
  Divide/1 -> [alpha]
  Constant/1 -> Divide/1
  Saturation/1 -> Divide/2
  speed_max/1 -> Abs/1
  Abs/1 -> Gain/1, Mux/2
  Gain/1 -> Mux/1
  Mux/1 -> MATLAB Function2/3(v)

== system ADRC_Toolbox/Advanced Motor Control/TD/order3_LTD ==
  u : Inport
  freq : Inport  Port=2
  reset : Inport  Port=3
  Demux : Demux  Outputs=3
  State space with reset : $bdroot/Advanced Motor Control/Basic/State space with reset  SystemSampleTime=-1  VariantActivationTime=update diagram  AllowFlexibleInterface=on  Latency=0  AutoFrameSizeCalculation=off
  Terminator : Terminator
  Terminator1 : Terminator
  set matrix : MATLAB Function  TreatAsAtomicUnit=on
  set x0 : MATLAB Function  TreatAsAtomicUnit=on
  y : Outport  VectorParamsAs1DForOutWhenUnconnected=off
  dy : Outport  Port=2  VectorParamsAs1DForOutWhenUnconnected=off
  ddy : Outport  Port=3  VectorParamsAs1DForOutWhenUnconnected=off
  wires:
  set matrix/4(D) -> State space with reset/5
  set matrix/3(C) -> State space with reset/4
  freq/1 -> set matrix/1(freq)
  set matrix/1(A) -> State space with reset/2
  set matrix/2(B) -> State space with reset/3
  u/1 -> State space with reset/1, set x0/1(u)
  State space with reset/1 -> Demux/1
  Demux/1 -> y/1
  Demux/2 -> dy/1
  Demux/3 -> ddy/1
  State space with reset/2 -> Terminator/1
  State space with reset/3 -> Terminator1/1
  set x0/1(x0) -> State space with reset/6
  reset/1 -> State space with reset/7

== system ADRC_Toolbox/Advanced Motor Control/TD/order5_LTD  ==
  u : Inport
  freq : Inport  Port=2
  reset : Inport  Port=3
  Demux : Demux  Outputs=3
  State space with reset : $bdroot/Advanced Motor Control/Basic/State space with reset  SystemSampleTime=-1  VariantActivationTime=update diagram  AllowFlexibleInterface=on  Latency=0  AutoFrameSizeCalculation=off
  Terminator : Terminator
  Terminator1 : Terminator
  set matrix : MATLAB Function  TreatAsAtomicUnit=on
  set x0 : MATLAB Function  TreatAsAtomicUnit=on
  y : Outport  VectorParamsAs1DForOutWhenUnconnected=off
  dy : Outport  Port=2  VectorParamsAs1DForOutWhenUnconnected=off
  ddy : Outport  Port=3  VectorParamsAs1DForOutWhenUnconnected=off
  wires:
  reset/1 -> State space with reset/7
  set x0/1(x0) -> State space with reset/6
  State space with reset/3 -> Terminator1/1
  State space with reset/2 -> Terminator/1
  Demux/3 -> ddy/1
  Demux/2 -> dy/1
  Demux/1 -> y/1
  State space with reset/1 -> Demux/1
  u/1 -> State space with reset/1, set x0/1(u)
  set matrix/2(B) -> State space with reset/3
  set matrix/1(A) -> State space with reset/2
  freq/1 -> set matrix/1(freq)
  set matrix/3(C) -> State space with reset/4
  set matrix/4(D) -> State space with reset/5

== system ADRC_Toolbox/Advanced Motor Control/TD/order7_LTD ==
  u : Inport
  freq : Inport  Port=2
  reset : Inport  Port=3
  Demux : Demux  Outputs=3
  State space with reset : $bdroot/Advanced Motor Control/Basic/State space with reset  SystemSampleTime=-1  VariantActivationTime=update diagram  AllowFlexibleInterface=on  Latency=0  AutoFrameSizeCalculation=off
  Terminator : Terminator
  Terminator1 : Terminator
  set matrix : MATLAB Function  TreatAsAtomicUnit=on
  set x0 : MATLAB Function  TreatAsAtomicUnit=on
  y : Outport  VectorParamsAs1DForOutWhenUnconnected=off
  dy : Outport  Port=2  VectorParamsAs1DForOutWhenUnconnected=off
  ddy : Outport  Port=3  VectorParamsAs1DForOutWhenUnconnected=off
  wires:
  set matrix/4(D) -> State space with reset/5
  set matrix/3(C) -> State space with reset/4
  freq/1 -> set matrix/1(freq)
  set matrix/1(A) -> State space with reset/2
  set matrix/2(B) -> State space with reset/3
  u/1 -> State space with reset/1, set x0/1(u)
  State space with reset/1 -> Demux/1
  Demux/1 -> y/1
  Demux/2 -> dy/1
  Demux/3 -> ddy/1
  State space with reset/2 -> Terminator/1
  State space with reset/3 -> Terminator1/1
  set x0/1(x0) -> State space with reset/6
  reset/1 -> State space with reset/7

== system ADRC_Toolbox/Advanced Motor Control/TD/order9_LTD ==
  u : Inport
  freq : Inport  Port=2
  reset : Inport  Port=3
  Demux : Demux  Outputs=3
  State space with reset : $bdroot/Advanced Motor Control/Basic/State space with reset  SystemSampleTime=-1  VariantActivationTime=update diagram  AllowFlexibleInterface=on  Latency=0  AutoFrameSizeCalculation=off
  Terminator : Terminator
  Terminator1 : Terminator
  set matrix : MATLAB Function  TreatAsAtomicUnit=on
  set x0 : MATLAB Function  TreatAsAtomicUnit=on
  y : Outport  VectorParamsAs1DForOutWhenUnconnected=off
  dy : Outport  Port=2  VectorParamsAs1DForOutWhenUnconnected=off
  ddy : Outport  Port=3  VectorParamsAs1DForOutWhenUnconnected=off
  wires:
  reset/1 -> State space with reset/7
  set x0/1(x0) -> State space with reset/6
  State space with reset/3 -> Terminator1/1
  State space with reset/2 -> Terminator/1
  Demux/3 -> ddy/1
  Demux/2 -> dy/1
  Demux/1 -> y/1
  State space with reset/1 -> Demux/1
  u/1 -> State space with reset/1, set x0/1(u)
  set matrix/2(B) -> State space with reset/3
  set matrix/1(A) -> State space with reset/2
  freq/1 -> set matrix/1(freq)
  set matrix/3(C) -> State space with reset/4
  set matrix/4(D) -> State space with reset/5

== matlab function ADRC_Toolbox/Interface/checkToolTypeMatched ==
  data: Arm_ToolType input; ErrorCode output; GeneralToolType input
function ErrorCode = checkToolTypeMatched(Arm_ToolType, GeneralToolType)
[~, ErrorCode] = isToolTypeMatched(Arm_ToolType, GeneralToolType);
end

== matlab function ADRC_Toolbox/Advanced Motor Control/Basic/ODE4 Continue State space/MATLAB Function ==
  data: A input; x_ output; B input; Ts input; x input; u input
function x_ = fcn(A,B,Ts,x, u)
w1 = x;
s1 = A*w1+B*u;
w2 = x + Ts/2*s1;
s2 = A*w2+B*u;
w3 = x + Ts/2*s2;
s3 = A*w3+B*u;
w4 = x + Ts*s3;
s4 = A*w4+B*u;

x_ = x + Ts/6*(s1 + 2*s2 + 2*s3 + s4);

== matlab function ADRC_Toolbox/Advanced Motor Control/Controller/2nd order Discrete LADRC/MATLAB Function2 ==
  data: wo input; b0 input; G output; H output; C output; D output; Ts parameter size=1
function [G, H, C, D] = C2D_zoh(wo, b0, Ts)

B = [0 3*wo;b0 3*wo^2 ; 0 wo^3 ];

G = [[ exp(-Ts*wo) + (Ts^2*wo^2*exp(-Ts*wo))/2 - 2*Ts*wo*exp(-Ts*wo),                Ts*exp(-Ts*wo) - (Ts^2*wo*exp(-Ts*wo))/2,                                        (Ts^2*exp(-Ts*wo))/2];
[                 Ts^2*wo^3*exp(-Ts*wo) - 3*Ts*wo^2*exp(-Ts*wo), exp(-Ts*wo) - Ts^2*wo^2*exp(-Ts*wo) + Ts*wo*exp(-Ts*wo),                        Ts*exp(-Ts*wo) + Ts^2*wo*exp(-Ts*wo)];
[               (Ts^2*wo^4*exp(-Ts*wo))/2 - Ts*wo^3*exp(-Ts*wo),                              -(Ts^2*wo^3*exp(-Ts*wo))/2, exp(-Ts*wo) + (Ts^2*wo^2*exp(-Ts*wo))/2 + Ts*wo*exp(-Ts*wo)];];

H = [[                             -(Ts*exp(-Ts*wo)*(Ts*wo - 2))/2,                          (Ts^2*exp(-Ts*wo))/2,            1/wo^3 - (exp(-Ts*wo)*(Ts^2*wo^2 + 2*Ts*wo + 2))/(2*wo^3)];
[ exp(-Ts*wo) - Ts^2*wo^2*exp(-Ts*wo) + Ts*wo*exp(-Ts*wo) - 1,                    Ts*exp(-Ts*wo)*(Ts*wo + 1),         -(exp(-Ts*wo)*(3*Ts*wo - 3*exp(Ts*wo) + Ts^2*wo^2 + 3))/wo^2];
[                                  -(Ts^2*wo^3*exp(-Ts*wo))/2, (exp(-Ts*wo)*(Ts^2*wo^2 + 2*Ts*wo + 2))/2 - 1, (3*exp(-Ts*wo)*(exp(Ts*wo) - 1))/wo - (Ts*exp(-Ts*wo)*(Ts*wo + 4))/2];]*B;
C = eye(3);
D = zeros(3,2);
end

== matlab function ADRC_Toolbox/Advanced Motor Control/Controller/2nd order LADRC/1//b1 ==
  data: u input; out output; b0 input
function out = b0(u, b0)
epsi = 1e-8;
if b0 < epsi
    out = 0;
else
    out = u/b0;
end

== matlab function ADRC_Toolbox/Advanced Motor Control/Controller/2nd order LADRC/MATLAB Function ==
  data: y input; x0 output
function x0 = init(y)
x0 = [y; 0; 0];
end

== matlab function ADRC_Toolbox/tools/Normal Tool Tmatrix ==
  data: theta_motor input size=14; T output size=[4,4]; P input Bus: Config_NormalTool_Bus size=1; open output size=1
function [T, open] = NormalTool_T(theta_motor, P)
% body = theta_motor(1:5);
arm = theta_motor(6:9);
MD = theta_motor(10:14);

screw = build_NormalTool(P);
[theta_joint, open] = screw.MDMotor2EndTool(arm, MD);

T = screw.FK(theta_joint);
end

== matlab function ADRC_Toolbox/utils/Tform2p ==
  data: T input; p output
function p = T2p(T)
p = T(1:3, 4);

== matlab function ADRC_Toolbox/Advanced Motor Control/Controller/2nd order LADRC/MATLAB Function1 ==
  data: wo input; A output; b0 input; B output; C output; D output
function [A, B, C, D] = fcn(wo, b0)
A = [-3*wo 1 0;-3*wo^2 0 1;-wo^3 0 0];
B = [0 3*wo;b0 3*wo^2 ; 0 wo^3 ];
C = eye(3);
D = zeros(3,2);

== matlab function ADRC_Toolbox/tools/Scope Tmatrix ==
  data: theta_motor input size=14; T output size=[4,4]; P input Bus: Config_Scope_Bus size=1; open output size=1; theta5 output
function [T, open, theta5] = Scope_T(theta_motor, P)
% body = theta_motor(1:5);
arm = theta_motor(6:9);
MD = theta_motor(10:14);

screw = build_Laparoscopy(P);
[theta_joint, open] = screw.MDMotor2EndTool(arm, MD);

T = screw.FK(theta_joint);
theta5 = theta_joint(end);
end

== matlab function ADRC_Toolbox/tools/Clamp Tmatrix ==
  data: theta_motor input size=14; T output size=[4,4]; P input Bus: Config_Clamp_Bus size=1; open output size=1
function [T, open] = Clamp_T(theta_motor, P)
% body = theta_motor(1:5);
arm = theta_motor(6:9);
MD = theta_motor(10:14);

screw = build_Clamp(P);
[theta_joint, open] = screw.MDMotor2EndTool(arm, MD);

T = screw.FK(theta_joint);
end

== matlab function ADRC_Toolbox/Advanced Motor Control/Controller/2nd order Discrete LADRC/1//b0 ==
  data: u input; out output; b0 input
function out = b0(u, b0)
epsi = 1e-8;
if b0 < epsi
    out = 0;
else
    out = u/b0;
end

== matlab function ADRC_Toolbox/Interface/physical2encoder_SC ==
  data: SC_physical input Bus: Hand_Bus size=1; SC_encoder output Bus: Hand_Bus size=1
function SC_encoder  = p2e_SC(SC_physical)

SC_encoder = physical2encoder_SC(SC_physical);
end

== matlab function ADRC_Toolbox/Advanced Motor Control/Controller/2nd order LADRC/derr_Kd1 ==
  data: u input; out output; wc input
function out = kd(u, wc)

out = u * wc * 2;

== matlab function ADRC_Toolbox/tools/Knife Tmatrix ==
  data: theta_motor input size=14; T output size=[4,4]; P input Bus: Config_Knife_Bus size=1; open output size=1; theta5 output
function [T, open, theta5] = knife_T(theta_motor, P)
% body = theta_motor(1:5);
arm = theta_motor(6:9);
MD = theta_motor(10:14);

screw = build_Knife(P);
[theta_joint, open] = screw.MDMotor2EndTool(arm, MD);
theta5 = theta_joint(end);
T = screw.FK(theta_joint);

end

== matlab function ADRC_Toolbox/Advanced Motor Control/Controller/2nd order Discrete LADRC/derr_Kd ==
  data: u input; out output; wc input
function out = kd(u, wc)

out = u * wc * 2;

== matlab function ADRC_Toolbox/Advanced Motor Control/Controller/2nd order Discrete LADRC/err_Kp ==
  data: u input; out output; wc input
function out = kp(u, wc)

out = u * wc^2;

== matlab function ADRC_Toolbox/Advanced Motor Control/Controller/2nd order Discrete LADRC/MATLAB Function ==
  data: y input; x0 output
function x0 = init(y)
x0 = [y; 0; 0];
end

== matlab function ADRC_Toolbox/Advanced Motor Control/Controller/2nd order LADRC/err_Kp1 ==
  data: u input; out output; wc input
function out = kp(u, wc)

out = u * wc^2;

== matlab function ADRC_Toolbox/Advanced Motor Control/Controller/2nd order MC-ADRC/1//b1 ==
  data: u input; out output; b0 input
function out = b0(u, b0)
epsi = 1e-8;
if b0 < epsi
    out = 0;
else
    out = u/b0;
end

== matlab function ADRC_Toolbox/Advanced Motor Control/Controller/2nd order MC-ADRC/MATLAB Function ==
  data: y input; x0 output
function x0 = init(y)
x0 = [y; 0; 0];
end

== matlab function ADRC_Toolbox/Advanced Motor Control/Controller/2nd order MC-ADRC/MATLAB Function1 ==
  data: wo input; A output; b0 input; B output; C output; D output; a1 input
function [A, B, C, D] = fcn(wo, b0, a1)
L1 = 3*wo - a1;
L2 = 3*wo^2 - L1*a1;
L3 = wo^3 - L2*a1;
A = [-L1 1 0;-L2 0 1;-L3 0 -a1];
B = [0 L1;b0 L2 ; -a1*b0 L3];
C = eye(3);
D = zeros(3,2);

== matlab function ADRC_Toolbox/Interface/encoder2physical_SC ==
  data: SC_encoder input Bus: Hand_Bus size=1; SC_physical output Bus: Hand_Bus size=1
function SC_physical  = e2p_SC(SC_encoder)

SC_physical = encoder2physical_SC(SC_encoder);
end

== matlab function ADRC_Toolbox/Advanced Motor Control/TD/order2_LTD with damping/set matrix ==
  data: freq input size=1; A output; B output; C output; D output; xi input
function [A,B,C,D] = fcn(freq, xi)
N = 2; % 阶数
wc = 2*pi*freq;
w = wc / sqrt(2^(1/N) - 1); 

wn = w;
A = [0, 1; -wn^2, -2*xi*wn];
B = zeros(2,1);
B(2) = wn^2;
C = eye(2);
D = 0;
end

== matlab function ADRC_Toolbox/Advanced Motor Control/Controller/2nd order MC-ADRC/derr_Kd1 ==
  data: u input; out output; wc input
function out = kd(u, wc)

out = u * wc * 2;

== matlab function ADRC_Toolbox/Advanced Motor Control/Controller/2nd order MC-ADRC/err_Kp1 ==
  data: u input; out output; wc input
function out = kp(u, wc)

out = u * wc^2;

== matlab function ADRC_Toolbox/Advanced Motor Control/TD/order2_LTD with damping/set x0 ==
  data: u input double size=1; x0 output double
function x0 = set_x0(u)
N = 2; %阶数
x0 = zeros(N,1);
x0(1) = u;

== matlab function ADRC_Toolbox/Advanced Motor Control/TD/LTD template/set matrix ==
  data: freq input size=1; A output; B output; C output; D output
function [A,B,C,D] = fcn(freq)
N = 5; % 阶数
wc = 2*pi*freq;
w = wc / sqrt(2^(1/N) - 1); 
A = zeros(N,N);
for k = 1:N-1
    A(k, k+1) = 1;
end
for k = 1:N
    A(N, k) = -nchoosek(N,k-1) * w^(N-k+1) ;
end
B = zeros(N,1);
B(N) = w^N;
C = zeros(3,N);
C(1,1) = 1;
C(2,2) = 1;
C(3,3) = 1;
D = 0;
end

== matlab function ADRC_Toolbox/Advanced Motor Control/TD/LTD template/set x0 ==
  data: u input double size=1; x0 output double
function x0 = set_x0(u)
N = 5; %阶数
x0 = zeros(N,1);
x0(1) = u;
